simulink model "modelsim"  (R2025a)
settings: Solver=ode23t  StartTime=0.0  StopTime=10.0  MaxStep=0.01  RelTol=1e-3
undefined symbols (not defined in the file or in its folder): X, Y, Z
libraries: sm_lib x91, nesl_utility x20, slpidlib x1
(part 3 of 3)

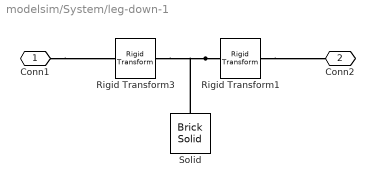
== system modelsim/System/leg-down-1 ==
  Rigid Transform1 : sm_lib/Frames and Transforms/Rigid Transform  RotationMethod=None  FollAlignAxisA=+X  BaseAlignAxisA=+Y  FollAlignAxisB=+Y  BaseAlignAxisB=+Z  RotationStandardAxis=+Z  RotationAngle=0.0  RotationAngleUnits=deg  RotationArbitraryAxis=[0 0 1]  RotationSequenceAxes=FollowerAxes  RotationSequence=XYX  RotationSequenceAngles=[0 0 0]  RotationSequenceAnglesUnits=deg  RotationMatrix=[1 0 0; 0 1 0; 0 0 1]  Quaternion=[1 0 0 0]  TranslationMethod=StandardAxis  TranslationCartesianOffset=[0 0 0]  TranslationCartesianOffsetUnits=m  TranslationStandardAxis=+X  TranslationStandardOffset=L/2  TranslationStandardOffsetUnits=m  TranslationROffset=0  TranslationROffsetUnits=m  TranslationThetaOffset=0  TranslationThetaOffsetUnits=deg  TranslationZOffset=0  TranslationZOffsetUnits=m
  Rigid Transform3 : sm_lib/Frames and Transforms/Rigid Transform  RotationMethod=None  FollAlignAxisA=+X  BaseAlignAxisA=+Y  FollAlignAxisB=+Y  BaseAlignAxisB=+Z  RotationStandardAxis=+Z  RotationAngle=0.0  RotationAngleUnits=deg  RotationArbitraryAxis=[0 0 1]  RotationSequenceAxes=FollowerAxes  RotationSequence=XYX  RotationSequenceAngles=[0 0 0]  RotationSequenceAnglesUnits=deg  RotationMatrix=[1 0 0; 0 1 0; 0 0 1]  Quaternion=[1 0 0 0]  TranslationMethod=StandardAxis  TranslationCartesianOffset=[0 0 0]  TranslationCartesianOffsetUnits=m  TranslationStandardAxis=+X  TranslationStandardOffset=L/2  TranslationStandardOffsetUnits=m  TranslationROffset=0  TranslationROffsetUnits=m  TranslationThetaOffset=0  TranslationThetaOffsetUnits=deg  TranslationZOffset=0  TranslationZOffsetUnits=m
  Solid : sm_lib/Body Elements/Brick Solid  BrickDimensions=[L H W]  BrickDimensionsUnits=m  ExportEntireGeometry=off  InertiaType=CalculateFromGeometry  BasedOnType=Density  Density=rho  DensityUnits=kg/m^3  Mass=1  MassUnits=kg  CenterOfMass=[0 0 0]  CenterOfMassUnits=m  MomentsOfInertia=[1 1 1]  MomentsOfInertiaUnits=kg*m^2  ProductsOfInertia=[0 0 0]  ProductsOfInertiaUnits=kg*m^2  GraphicType=FromGeometry  MarkerShape=Sphere  MarkerSize=10  GraphicVisPropType=SimpleVisualProperties  GraphicDiffuseColor=[0.5 0.5 0.5]  GraphicOpacity=1.0  GraphicSpecularColor=[0.5 0.5 0.5 1.0]  GraphicAmbientColor=[0.15 0.15 0.15 1.0]  GraphicEmissiveColor=[0.0 0.0 0.0 1.0]  GraphicShininess=75  DoExposeReferenceFrame=on  SerializedFrames=<Frames/>
  Conn1 : PMIOPort  Side=Left
  Conn2 : PMIOPort  Port=2  Side=Right
  connections:
  Rigid Transform1/RConn1 -- Conn2/RConn1
  Conn1/RConn1 -- Rigid Transform3/LConn1
  Rigid Transform1/LConn1 -- Solid/RConn1 -- Rigid Transform3/RConn1

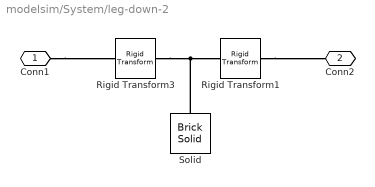
== system modelsim/System/leg-down-2 ==
  Rigid Transform1 : sm_lib/Frames and Transforms/Rigid Transform  RotationMethod=None  FollAlignAxisA=+X  BaseAlignAxisA=+Y  FollAlignAxisB=+Y  BaseAlignAxisB=+Z  RotationStandardAxis=+Z  RotationAngle=0.0  RotationAngleUnits=deg  RotationArbitraryAxis=[0 0 1]  RotationSequenceAxes=FollowerAxes  RotationSequence=XYX  RotationSequenceAngles=[0 0 0]  RotationSequenceAnglesUnits=deg  RotationMatrix=[1 0 0; 0 1 0; 0 0 1]  Quaternion=[1 0 0 0]  TranslationMethod=StandardAxis  TranslationCartesianOffset=[0 0 0]  TranslationCartesianOffsetUnits=m  TranslationStandardAxis=+X  TranslationStandardOffset=L/2  TranslationStandardOffsetUnits=m  TranslationROffset=0  TranslationROffsetUnits=m  TranslationThetaOffset=0  TranslationThetaOffsetUnits=deg  TranslationZOffset=0  TranslationZOffsetUnits=m
  Rigid Transform3 : sm_lib/Frames and Transforms/Rigid Transform  RotationMethod=None  FollAlignAxisA=+X  BaseAlignAxisA=+Y  FollAlignAxisB=+Y  BaseAlignAxisB=+Z  RotationStandardAxis=+Z  RotationAngle=0.0  RotationAngleUnits=deg  RotationArbitraryAxis=[0 0 1]  RotationSequenceAxes=FollowerAxes  RotationSequence=XYX  RotationSequenceAngles=[0 0 0]  RotationSequenceAnglesUnits=deg  RotationMatrix=[1 0 0; 0 1 0; 0 0 1]  Quaternion=[1 0 0 0]  TranslationMethod=StandardAxis  TranslationCartesianOffset=[0 0 0]  TranslationCartesianOffsetUnits=m  TranslationStandardAxis=+X  TranslationStandardOffset=L/2  TranslationStandardOffsetUnits=m  TranslationROffset=0  TranslationROffsetUnits=m  TranslationThetaOffset=0  TranslationThetaOffsetUnits=deg  TranslationZOffset=0  TranslationZOffsetUnits=m
  Solid : sm_lib/Body Elements/Brick Solid  BrickDimensions=[L H W]  BrickDimensionsUnits=m  ExportEntireGeometry=off  InertiaType=CalculateFromGeometry  BasedOnType=Density  Density=rho  DensityUnits=kg/m^3  Mass=1  MassUnits=kg  CenterOfMass=[0 0 0]  CenterOfMassUnits=m  MomentsOfInertia=[1 1 1]  MomentsOfInertiaUnits=kg*m^2  ProductsOfInertia=[0 0 0]  ProductsOfInertiaUnits=kg*m^2  GraphicType=FromGeometry  MarkerShape=Sphere  MarkerSize=10  GraphicVisPropType=SimpleVisualProperties  GraphicDiffuseColor=[0.5 0.5 0.5]  GraphicOpacity=1.0  GraphicSpecularColor=[0.5 0.5 0.5 1.0]  GraphicAmbientColor=[0.15 0.15 0.15 1.0]  GraphicEmissiveColor=[0.0 0.0 0.0 1.0]  GraphicShininess=75  DoExposeReferenceFrame=on  SerializedFrames=<Frames/>
  Conn1 : PMIOPort  Side=Left
  Conn2 : PMIOPort  Port=2  Side=Right
  connections:
  Rigid Transform3/RConn1 -- Solid/RConn1 -- Rigid Transform1/LConn1
  Conn1/RConn1 -- Rigid Transform3/LConn1
  Rigid Transform1/RConn1 -- Conn2/RConn1

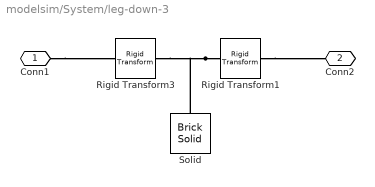
== system modelsim/System/leg-down-3 ==
  Rigid Transform1 : sm_lib/Frames and Transforms/Rigid Transform  RotationMethod=None  FollAlignAxisA=+X  BaseAlignAxisA=+Y  FollAlignAxisB=+Y  BaseAlignAxisB=+Z  RotationStandardAxis=+Z  RotationAngle=0.0  RotationAngleUnits=deg  RotationArbitraryAxis=[0 0 1]  RotationSequenceAxes=FollowerAxes  RotationSequence=XYX  RotationSequenceAngles=[0 0 0]  RotationSequenceAnglesUnits=deg  RotationMatrix=[1 0 0; 0 1 0; 0 0 1]  Quaternion=[1 0 0 0]  TranslationMethod=StandardAxis  TranslationCartesianOffset=[0 0 0]  TranslationCartesianOffsetUnits=m  TranslationStandardAxis=+X  TranslationStandardOffset=L/2  TranslationStandardOffsetUnits=m  TranslationROffset=0  TranslationROffsetUnits=m  TranslationThetaOffset=0  TranslationThetaOffsetUnits=deg  TranslationZOffset=0  TranslationZOffsetUnits=m
  Rigid Transform3 : sm_lib/Frames and Transforms/Rigid Transform  RotationMethod=None  FollAlignAxisA=+X  BaseAlignAxisA=+Y  FollAlignAxisB=+Y  BaseAlignAxisB=+Z  RotationStandardAxis=+Z  RotationAngle=0.0  RotationAngleUnits=deg  RotationArbitraryAxis=[0 0 1]  RotationSequenceAxes=FollowerAxes  RotationSequence=XYX  RotationSequenceAngles=[0 0 0]  RotationSequenceAnglesUnits=deg  RotationMatrix=[1 0 0; 0 1 0; 0 0 1]  Quaternion=[1 0 0 0]  TranslationMethod=StandardAxis  TranslationCartesianOffset=[0 0 0]  TranslationCartesianOffsetUnits=m  TranslationStandardAxis=+X  TranslationStandardOffset=L/2  TranslationStandardOffsetUnits=m  TranslationROffset=0  TranslationROffsetUnits=m  TranslationThetaOffset=0  TranslationThetaOffsetUnits=deg  TranslationZOffset=0  TranslationZOffsetUnits=m
  Solid : sm_lib/Body Elements/Brick Solid  BrickDimensions=[L H W]  BrickDimensionsUnits=m  ExportEntireGeometry=off  InertiaType=CalculateFromGeometry  BasedOnType=Density  Density=rho  DensityUnits=kg/m^3  Mass=1  MassUnits=kg  CenterOfMass=[0 0 0]  CenterOfMassUnits=m  MomentsOfInertia=[1 1 1]  MomentsOfInertiaUnits=kg*m^2  ProductsOfInertia=[0 0 0]  ProductsOfInertiaUnits=kg*m^2  GraphicType=FromGeometry  MarkerShape=Sphere  MarkerSize=10  GraphicVisPropType=SimpleVisualProperties  GraphicDiffuseColor=[0.5 0.5 0.5]  GraphicOpacity=1.0  GraphicSpecularColor=[0.5 0.5 0.5 1.0]  GraphicAmbientColor=[0.15 0.15 0.15 1.0]  GraphicEmissiveColor=[0.0 0.0 0.0 1.0]  GraphicShininess=75  DoExposeReferenceFrame=on  SerializedFrames=<Frames/>
  Conn1 : PMIOPort  Side=Left
  Conn2 : PMIOPort  Port=2  Side=Right
  connections:
  Rigid Transform1/RConn1 -- Conn2/RConn1
  Conn1/RConn1 -- Rigid Transform3/LConn1
  Rigid Transform1/LConn1 -- Solid/RConn1 -- Rigid Transform3/RConn1

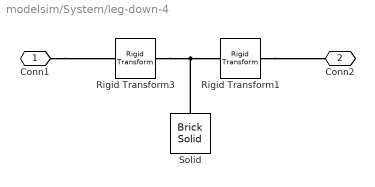
== system modelsim/System/leg-down-4 ==
  Rigid Transform1 : sm_lib/Frames and Transforms/Rigid Transform  RotationMethod=None  FollAlignAxisA=+X  BaseAlignAxisA=+Y  FollAlignAxisB=+Y  BaseAlignAxisB=+Z  RotationStandardAxis=+Z  RotationAngle=0.0  RotationAngleUnits=deg  RotationArbitraryAxis=[0 0 1]  RotationSequenceAxes=FollowerAxes  RotationSequence=XYX  RotationSequenceAngles=[0 0 0]  RotationSequenceAnglesUnits=deg  RotationMatrix=[1 0 0; 0 1 0; 0 0 1]  Quaternion=[1 0 0 0]  TranslationMethod=StandardAxis  TranslationCartesianOffset=[0 0 0]  TranslationCartesianOffsetUnits=m  TranslationStandardAxis=+X  TranslationStandardOffset=L/2  TranslationStandardOffsetUnits=m  TranslationROffset=0  TranslationROffsetUnits=m  TranslationThetaOffset=0  TranslationThetaOffsetUnits=deg  TranslationZOffset=0  TranslationZOffsetUnits=m
  Rigid Transform3 : sm_lib/Frames and Transforms/Rigid Transform  RotationMethod=None  FollAlignAxisA=+X  BaseAlignAxisA=+Y  FollAlignAxisB=+Y  BaseAlignAxisB=+Z  RotationStandardAxis=+Z  RotationAngle=0.0  RotationAngleUnits=deg  RotationArbitraryAxis=[0 0 1]  RotationSequenceAxes=FollowerAxes  RotationSequence=XYX  RotationSequenceAngles=[0 0 0]  RotationSequenceAnglesUnits=deg  RotationMatrix=[1 0 0; 0 1 0; 0 0 1]  Quaternion=[1 0 0 0]  TranslationMethod=StandardAxis  TranslationCartesianOffset=[0 0 0]  TranslationCartesianOffsetUnits=m  TranslationStandardAxis=+X  TranslationStandardOffset=L/2  TranslationStandardOffsetUnits=m  TranslationROffset=0  TranslationROffsetUnits=m  TranslationThetaOffset=0  TranslationThetaOffsetUnits=deg  TranslationZOffset=0  TranslationZOffsetUnits=m
  Solid : sm_lib/Body Elements/Brick Solid  BrickDimensions=[L H W]  BrickDimensionsUnits=m  ExportEntireGeometry=off  InertiaType=CalculateFromGeometry  BasedOnType=Density  Density=rho  DensityUnits=kg/m^3  Mass=1  MassUnits=kg  CenterOfMass=[0 0 0]  CenterOfMassUnits=m  MomentsOfInertia=[1 1 1]  MomentsOfInertiaUnits=kg*m^2  ProductsOfInertia=[0 0 0]  ProductsOfInertiaUnits=kg*m^2  GraphicType=FromGeometry  MarkerShape=Sphere  MarkerSize=10  GraphicVisPropType=SimpleVisualProperties  GraphicDiffuseColor=[0.5 0.5 0.5]  GraphicOpacity=1.0  GraphicSpecularColor=[0.5 0.5 0.5 1.0]  GraphicAmbientColor=[0.15 0.15 0.15 1.0]  GraphicEmissiveColor=[0.0 0.0 0.0 1.0]  GraphicShininess=75  DoExposeReferenceFrame=on  SerializedFrames=<Frames/>
  Conn1 : PMIOPort  Side=Left
  Conn2 : PMIOPort  Port=2  Side=Right
  connections:
  Rigid Transform3/RConn1 -- Solid/RConn1 -- Rigid Transform1/LConn1
  Conn1/RConn1 -- Rigid Transform3/LConn1
  Rigid Transform1/RConn1 -- Conn2/RConn1

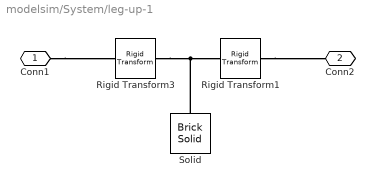
== system modelsim/System/leg-up-1 ==
  Rigid Transform1 : sm_lib/Frames and Transforms/Rigid Transform  RotationMethod=None  FollAlignAxisA=+X  BaseAlignAxisA=+Y  FollAlignAxisB=+Y  BaseAlignAxisB=+Z  RotationStandardAxis=+Z  RotationAngle=0.0  RotationAngleUnits=deg  RotationArbitraryAxis=[0 0 1]  RotationSequenceAxes=FollowerAxes  RotationSequence=XYX  RotationSequenceAngles=[0 0 0]  RotationSequenceAnglesUnits=deg  RotationMatrix=[1 0 0; 0 1 0; 0 0 1]  Quaternion=[1 0 0 0]  TranslationMethod=StandardAxis  TranslationCartesianOffset=[0 0 0]  TranslationCartesianOffsetUnits=m  TranslationStandardAxis=+X  TranslationStandardOffset=L/2  TranslationStandardOffsetUnits=m  TranslationROffset=0  TranslationROffsetUnits=m  TranslationThetaOffset=0  TranslationThetaOffsetUnits=deg  TranslationZOffset=0  TranslationZOffsetUnits=m
  Rigid Transform3 : sm_lib/Frames and Transforms/Rigid Transform  RotationMethod=None  FollAlignAxisA=+X  BaseAlignAxisA=+Y  FollAlignAxisB=+Y  BaseAlignAxisB=+Z  RotationStandardAxis=+Z  RotationAngle=0.0  RotationAngleUnits=deg  RotationArbitraryAxis=[0 0 1]  RotationSequenceAxes=FollowerAxes  RotationSequence=XYX  RotationSequenceAngles=[0 0 0]  RotationSequenceAnglesUnits=deg  RotationMatrix=[1 0 0; 0 1 0; 0 0 1]  Quaternion=[1 0 0 0]  TranslationMethod=StandardAxis  TranslationCartesianOffset=[0 0 0]  TranslationCartesianOffsetUnits=m  TranslationStandardAxis=+X  TranslationStandardOffset=L/2  TranslationStandardOffsetUnits=m  TranslationROffset=0  TranslationROffsetUnits=m  TranslationThetaOffset=0  TranslationThetaOffsetUnits=deg  TranslationZOffset=0  TranslationZOffsetUnits=m
  Solid : sm_lib/Body Elements/Brick Solid  BrickDimensions=[L H W]  BrickDimensionsUnits=m  ExportEntireGeometry=off  InertiaType=CalculateFromGeometry  BasedOnType=Density  Density=rho  DensityUnits=kg/m^3  Mass=1  MassUnits=kg  CenterOfMass=[0 0 0]  CenterOfMassUnits=m  MomentsOfInertia=[1 1 1]  MomentsOfInertiaUnits=kg*m^2  ProductsOfInertia=[0 0 0]  ProductsOfInertiaUnits=kg*m^2  GraphicType=FromGeometry  MarkerShape=Sphere  MarkerSize=10  GraphicVisPropType=SimpleVisualProperties  GraphicDiffuseColor=[0.5 0.5 0.5]  GraphicOpacity=1.0  GraphicSpecularColor=[0.5 0.5 0.5 1.0]  GraphicAmbientColor=[0.15 0.15 0.15 1.0]  GraphicEmissiveColor=[0.0 0.0 0.0 1.0]  GraphicShininess=75  DoExposeReferenceFrame=on  SerializedFrames=<Frames/>
  Conn1 : PMIOPort  Side=Left
  Conn2 : PMIOPort  Port=2  Side=Right
  connections:
  Solid/RConn1 -- Rigid Transform3/RConn1 -- Rigid Transform1/LConn1
  Conn1/RConn1 -- Rigid Transform3/LConn1
  Rigid Transform1/RConn1 -- Conn2/RConn1

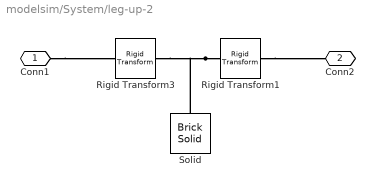
== system modelsim/System/leg-up-2 ==
  Rigid Transform1 : sm_lib/Frames and Transforms/Rigid Transform  RotationMethod=None  FollAlignAxisA=+X  BaseAlignAxisA=+Y  FollAlignAxisB=+Y  BaseAlignAxisB=+Z  RotationStandardAxis=+Z  RotationAngle=0.0  RotationAngleUnits=deg  RotationArbitraryAxis=[0 0 1]  RotationSequenceAxes=FollowerAxes  RotationSequence=XYX  RotationSequenceAngles=[0 0 0]  RotationSequenceAnglesUnits=deg  RotationMatrix=[1 0 0; 0 1 0; 0 0 1]  Quaternion=[1 0 0 0]  TranslationMethod=StandardAxis  TranslationCartesianOffset=[0 0 0]  TranslationCartesianOffsetUnits=m  TranslationStandardAxis=+X  TranslationStandardOffset=L/2  TranslationStandardOffsetUnits=m  TranslationROffset=0  TranslationROffsetUnits=m  TranslationThetaOffset=0  TranslationThetaOffsetUnits=deg  TranslationZOffset=0  TranslationZOffsetUnits=m
  Rigid Transform3 : sm_lib/Frames and Transforms/Rigid Transform  RotationMethod=None  FollAlignAxisA=+X  BaseAlignAxisA=+Y  FollAlignAxisB=+Y  BaseAlignAxisB=+Z  RotationStandardAxis=+Z  RotationAngle=0.0  RotationAngleUnits=deg  RotationArbitraryAxis=[0 0 1]  RotationSequenceAxes=FollowerAxes  RotationSequence=XYX  RotationSequenceAngles=[0 0 0]  RotationSequenceAnglesUnits=deg  RotationMatrix=[1 0 0; 0 1 0; 0 0 1]  Quaternion=[1 0 0 0]  TranslationMethod=StandardAxis  TranslationCartesianOffset=[0 0 0]  TranslationCartesianOffsetUnits=m  TranslationStandardAxis=+X  TranslationStandardOffset=L/2  TranslationStandardOffsetUnits=m  TranslationROffset=0  TranslationROffsetUnits=m  TranslationThetaOffset=0  TranslationThetaOffsetUnits=deg  TranslationZOffset=0  TranslationZOffsetUnits=m
  Solid : sm_lib/Body Elements/Brick Solid  BrickDimensions=[L H W]  BrickDimensionsUnits=m  ExportEntireGeometry=off  InertiaType=CalculateFromGeometry  BasedOnType=Density  Density=rho  DensityUnits=kg/m^3  Mass=1  MassUnits=kg  CenterOfMass=[0 0 0]  CenterOfMassUnits=m  MomentsOfInertia=[1 1 1]  MomentsOfInertiaUnits=kg*m^2  ProductsOfInertia=[0 0 0]  ProductsOfInertiaUnits=kg*m^2  GraphicType=FromGeometry  MarkerShape=Sphere  MarkerSize=10  GraphicVisPropType=SimpleVisualProperties  GraphicDiffuseColor=[0.5 0.5 0.5]  GraphicOpacity=1.0  GraphicSpecularColor=[0.5 0.5 0.5 1.0]  GraphicAmbientColor=[0.15 0.15 0.15 1.0]  GraphicEmissiveColor=[0.0 0.0 0.0 1.0]  GraphicShininess=75  DoExposeReferenceFrame=on  SerializedFrames=<Frames/>
  Conn1 : PMIOPort  Side=Left
  Conn2 : PMIOPort  Port=2  Side=Right
  connections:
  Rigid Transform1/RConn1 -- Conn2/RConn1
  Conn1/RConn1 -- Rigid Transform3/LConn1
  Rigid Transform1/LConn1 -- Solid/RConn1 -- Rigid Transform3/RConn1

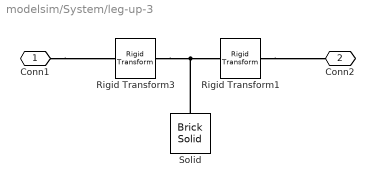
== system modelsim/System/leg-up-3 ==
  Rigid Transform1 : sm_lib/Frames and Transforms/Rigid Transform  RotationMethod=None  FollAlignAxisA=+X  BaseAlignAxisA=+Y  FollAlignAxisB=+Y  BaseAlignAxisB=+Z  RotationStandardAxis=+Z  RotationAngle=0.0  RotationAngleUnits=deg  RotationArbitraryAxis=[0 0 1]  RotationSequenceAxes=FollowerAxes  RotationSequence=XYX  RotationSequenceAngles=[0 0 0]  RotationSequenceAnglesUnits=deg  RotationMatrix=[1 0 0; 0 1 0; 0 0 1]  Quaternion=[1 0 0 0]  TranslationMethod=StandardAxis  TranslationCartesianOffset=[0 0 0]  TranslationCartesianOffsetUnits=m  TranslationStandardAxis=+X  TranslationStandardOffset=L/2  TranslationStandardOffsetUnits=m  TranslationROffset=0  TranslationROffsetUnits=m  TranslationThetaOffset=0  TranslationThetaOffsetUnits=deg  TranslationZOffset=0  TranslationZOffsetUnits=m
  Rigid Transform3 : sm_lib/Frames and Transforms/Rigid Transform  RotationMethod=None  FollAlignAxisA=+X  BaseAlignAxisA=+Y  FollAlignAxisB=+Y  BaseAlignAxisB=+Z  RotationStandardAxis=+Z  RotationAngle=0.0  RotationAngleUnits=deg  RotationArbitraryAxis=[0 0 1]  RotationSequenceAxes=FollowerAxes  RotationSequence=XYX  RotationSequenceAngles=[0 0 0]  RotationSequenceAnglesUnits=deg  RotationMatrix=[1 0 0; 0 1 0; 0 0 1]  Quaternion=[1 0 0 0]  TranslationMethod=StandardAxis  TranslationCartesianOffset=[0 0 0]  TranslationCartesianOffsetUnits=m  TranslationStandardAxis=+X  TranslationStandardOffset=L/2  TranslationStandardOffsetUnits=m  TranslationROffset=0  TranslationROffsetUnits=m  TranslationThetaOffset=0  TranslationThetaOffsetUnits=deg  TranslationZOffset=0  TranslationZOffsetUnits=m
  Solid : sm_lib/Body Elements/Brick Solid  BrickDimensions=[L H W]  BrickDimensionsUnits=m  ExportEntireGeometry=off  InertiaType=CalculateFromGeometry  BasedOnType=Density  Density=rho  DensityUnits=kg/m^3  Mass=1  MassUnits=kg  CenterOfMass=[0 0 0]  CenterOfMassUnits=m  MomentsOfInertia=[1 1 1]  MomentsOfInertiaUnits=kg*m^2  ProductsOfInertia=[0 0 0]  ProductsOfInertiaUnits=kg*m^2  GraphicType=FromGeometry  MarkerShape=Sphere  MarkerSize=10  GraphicVisPropType=SimpleVisualProperties  GraphicDiffuseColor=[0.5 0.5 0.5]  GraphicOpacity=1.0  GraphicSpecularColor=[0.5 0.5 0.5 1.0]  GraphicAmbientColor=[0.15 0.15 0.15 1.0]  GraphicEmissiveColor=[0.0 0.0 0.0 1.0]  GraphicShininess=75  DoExposeReferenceFrame=on  SerializedFrames=<Frames/>
  Conn1 : PMIOPort  Side=Left
  Conn2 : PMIOPort  Port=2  Side=Right
  connections:
  Solid/RConn1 -- Rigid Transform3/RConn1 -- Rigid Transform1/LConn1
  Conn1/RConn1 -- Rigid Transform3/LConn1
  Rigid Transform1/RConn1 -- Conn2/RConn1

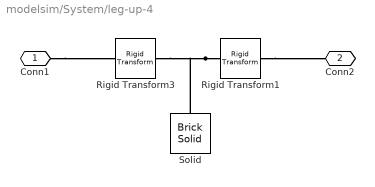
== system modelsim/System/leg-up-4 ==
  Rigid Transform1 : sm_lib/Frames and Transforms/Rigid Transform  RotationMethod=None  FollAlignAxisA=+X  BaseAlignAxisA=+Y  FollAlignAxisB=+Y  BaseAlignAxisB=+Z  RotationStandardAxis=+Z  RotationAngle=0.0  RotationAngleUnits=deg  RotationArbitraryAxis=[0 0 1]  RotationSequenceAxes=FollowerAxes  RotationSequence=XYX  RotationSequenceAngles=[0 0 0]  RotationSequenceAnglesUnits=deg  RotationMatrix=[1 0 0; 0 1 0; 0 0 1]  Quaternion=[1 0 0 0]  TranslationMethod=StandardAxis  TranslationCartesianOffset=[0 0 0]  TranslationCartesianOffsetUnits=m  TranslationStandardAxis=+X  TranslationStandardOffset=L/2  TranslationStandardOffsetUnits=m  TranslationROffset=0  TranslationROffsetUnits=m  TranslationThetaOffset=0  TranslationThetaOffsetUnits=deg  TranslationZOffset=0  TranslationZOffsetUnits=m
  Rigid Transform3 : sm_lib/Frames and Transforms/Rigid Transform  RotationMethod=None  FollAlignAxisA=+X  BaseAlignAxisA=+Y  FollAlignAxisB=+Y  BaseAlignAxisB=+Z  RotationStandardAxis=+Z  RotationAngle=0.0  RotationAngleUnits=deg  RotationArbitraryAxis=[0 0 1]  RotationSequenceAxes=FollowerAxes  RotationSequence=XYX  RotationSequenceAngles=[0 0 0]  RotationSequenceAnglesUnits=deg  RotationMatrix=[1 0 0; 0 1 0; 0 0 1]  Quaternion=[1 0 0 0]  TranslationMethod=StandardAxis  TranslationCartesianOffset=[0 0 0]  TranslationCartesianOffsetUnits=m  TranslationStandardAxis=+X  TranslationStandardOffset=L/2  TranslationStandardOffsetUnits=m  TranslationROffset=0  TranslationROffsetUnits=m  TranslationThetaOffset=0  TranslationThetaOffsetUnits=deg  TranslationZOffset=0  TranslationZOffsetUnits=m
  Solid : sm_lib/Body Elements/Brick Solid  BrickDimensions=[L H W]  BrickDimensionsUnits=m  ExportEntireGeometry=off  InertiaType=CalculateFromGeometry  BasedOnType=Density  Density=rho  DensityUnits=kg/m^3  Mass=1  MassUnits=kg  CenterOfMass=[0 0 0]  CenterOfMassUnits=m  MomentsOfInertia=[1 1 1]  MomentsOfInertiaUnits=kg*m^2  ProductsOfInertia=[0 0 0]  ProductsOfInertiaUnits=kg*m^2  GraphicType=FromGeometry  MarkerShape=Sphere  MarkerSize=10  GraphicVisPropType=SimpleVisualProperties  GraphicDiffuseColor=[0.5 0.5 0.5]  GraphicOpacity=1.0  GraphicSpecularColor=[0.5 0.5 0.5 1.0]  GraphicAmbientColor=[0.15 0.15 0.15 1.0]  GraphicEmissiveColor=[0.0 0.0 0.0 1.0]  GraphicShininess=75  DoExposeReferenceFrame=on  SerializedFrames=<Frames/>
  Conn1 : PMIOPort  Side=Left
  Conn2 : PMIOPort  Port=2  Side=Right
  connections:
  Rigid Transform1/RConn1 -- Conn2/RConn1
  Conn1/RConn1 -- Rigid Transform3/LConn1
  Rigid Transform1/LConn1 -- Solid/RConn1 -- Rigid Transform3/RConn1

== matlab function modelsim/MATLAB Function1 ==
  data: L output; phi0 output; phi1 input; xdot output; phi4 input; phi1dot input; phi4dot input
function [L,phi0,xdot] = vmcX(phi1,phi4,phi1dot,phi4dot)
%vmcX
%    [L,PHI0,XDOT] = vmcX(PHI1,PHI4,PHI1DOT,PHI4DOT)

%    This function was generated by the Symbolic Math Toolbox version 25.1.
%    2025-12-08 16:42:02

t2 = cos(phi1);
t3 = cos(phi4);
t4 = sin(phi1);
t5 = sin(phi4);
t6 = t2.*(3.0./2.0e+1);
t7 = t3.*(3.0./2.0e+1);
t8 = t4.*(3.0./2.0e+1);
t9 = t5.*(3.0./2.0e+1);
t12 = t4.*1.5e-1i;
t13 = t5.*1.5e-1i;
t15 = t2.*(8.1e+1./1.0e+3);
t16 = t3.*(8.1e+1./1.0e+3);
t17 = t4.*(8.1e+1./1.0e+3);
t18 = t5.*(8.1e+1./1.0e+3);
t21 = t4.*8.1e-2i;
t22 = t5.*8.1e-2i;
t10 = -t6;
t11 = -t9;
t14 = -t12;
t19 = -t15;
t20 = -t18;
t23 = -t21;
t24 = t8+t11;
t26 = t7+t10+3.0./2.0e+1;
t28 = t17+t20;
t30 = t16+t19+8.1e+1./1.0e+3;
t25 = t24.^2;
t27 = t26.^2;
t29 = t28.^2;
t31 = t30.^2;
t32 = t25+t27;
t33 = t32.^2;
t34 = -t33;
t35 = t29+t31+t34;
t36 = sqrt(t35);
t37 = t36.*1i;
t38 = t22+t23+t30+t32+t37;
t39 = angle(t38);
t40 = t39.*2.0;
t41 = -t40;
t42 = cos(t40);
t43 = sin(t40);
t44 = phi1+t41;
t45 = phi4+t41;
t48 = t42.*(2.7e+1./1.0e+2);
t49 = t43.*(2.7e+1./1.0e+2);
t51 = t43.*2.7e-1i;
t46 = sin(t44);
t47 = sin(t45);
t50 = -t48;
t52 = -t51;
t53 = t8+t49;
t55 = t6+t48-3.0./4.0e+1;
t54 = t53.^2;
t56 = t55.^2;
t57 = t12+t51+t55;
t64 = t13+t14+t26+t50+t52;
t58 = angle(t57);
t59 = t54+t56;
t65 = angle(t64);
t60 = -t58;
t63 = 1.0./sqrt(t59);
L = 1.0./t63;
if nargout > 1
    phi0 = t58;
end
if nargout > 2
    t66 = -t65;
    t61 = phi1+t60;
    t62 = phi4+t60;
    t67 = phi1+t66;
    t68 = phi4+t66;
    t71 = t40+t60;
    t74 = t40+t66;
    t77 = t60+t65;
    t69 = sin(t67);
    t70 = sin(t68);
    t72 = cos(t71);
    t73 = sin(t71);
    t75 = sin(t74);
    t78 = cos(t77);
    t79 = sin(t77);
    t76 = 1.0./t75;
    xdot = [phi1dot.*(sin(t61).*(-3.0./2.0e+1)+t46.*t76.*t79.*(3.0./2.0e+1)+t69.*t73.*t76.*(3.0./2.0e+1))-phi4dot.*(sin(t62).*(3.0./2.0e+1)+t47.*t76.*t79.*(3.0./2.0e+1)+t70.*t73.*t76.*(3.0./2.0e+1));-phi1dot.*t63.*(cos(t61).*(-3.0./2.0e+1)+t46.*t76.*t78.*(3.0./2.0e+1)+t69.*t72.*t76.*(3.0./2.0e+1))+phi4dot.*t63.*(cos(t62).*(3.0./2.0e+1)+t47.*t76.*t78.*(3.0./2.0e+1)+t70.*t72.*t76.*(3.0./2.0e+1))];
end
end

== matlab function modelsim/MATLAB Function ==
  data: F input; T output; Tp input; phi1 input; phi4 input
function T = vmcT(F,Tp,phi1,phi4)
%vmcT
%    T = vmcT(F,Tp,PHI1,PHI4)

%    This function was generated by the Symbolic Math Toolbox version 25.1.
%    2025-12-08 15:34:32

t2 = cos(phi1);
t3 = cos(phi4);
t4 = sin(phi1);
t5 = sin(phi4);
t6 = t2.*(3.0./2.0e+1);
t7 = t3.*(3.0./2.0e+1);
t8 = t4.*(3.0./2.0e+1);
t9 = t5.*(3.0./2.0e+1);
t12 = t4.*1.5e-1i;
t13 = t5.*1.5e-1i;
t15 = t2.*(8.1e+1./1.0e+3);
t16 = t3.*(8.1e+1./1.0e+3);
t17 = t4.*(8.1e+1./1.0e+3);
t18 = t5.*(8.1e+1./1.0e+3);
t21 = t4.*8.1e-2i;
t22 = t5.*8.1e-2i;
t10 = -t6;
t11 = -t9;
t14 = -t12;
t19 = -t15;
t20 = -t18;
t23 = -t21;
t24 = t8+t11;
t26 = t7+t10+3.0./2.0e+1;
t28 = t17+t20;
t30 = t16+t19+8.1e+1./1.0e+3;
t25 = t24.^2;
t27 = t26.^2;
t29 = t28.^2;
t31 = t30.^2;
t32 = t25+t27;
t33 = t32.^2;
t34 = -t33;
t35 = t29+t31+t34;
t36 = sqrt(t35);
t37 = t36.*1i;
t38 = t22+t23+t30+t32+t37;
t39 = angle(t38);
t40 = t39.*2.0;
t41 = -t40;
t42 = cos(t40);
t43 = sin(t40);
t44 = phi1+t41;
t45 = phi4+t41;
t48 = t42.*(2.7e+1./1.0e+2);
t49 = t43.*(2.7e+1./1.0e+2);
t51 = t43.*2.7e-1i;
t46 = sin(t44);
t47 = sin(t45);
t50 = -t48;
t52 = -t51;
t53 = t8+t49;
t55 = t6+t48-3.0./4.0e+1;
t54 = t53.^2;
t56 = t55.^2;
t57 = t12+t51+t55;
t64 = t13+t14+t26+t50+t52;
t58 = angle(t57);
t59 = t54+t56;
t65 = angle(t64);
t60 = -t58;
t63 = 1.0./sqrt(t59);
t66 = -t65;
t61 = phi1+t60;
t62 = phi4+t60;
t67 = phi1+t66;
t68 = phi4+t66;
t71 = t40+t60;
t74 = t40+t66;
t77 = t60+t65;
t69 = sin(t67);
t70 = sin(t68);
t72 = cos(t71);
t73 = sin(t71);
t75 = sin(t74);
t78 = cos(t77);
t79 = sin(t77);
t76 = 1.0./t75;
T = [F.*(sin(t61).*(-3.0./2.0e+1)+t46.*t76.*t79.*(3.0./2.0e+1)+t69.*t73.*t76.*(3.0./2.0e+1))-Tp.*t63.*(cos(t61).*(-3.0./2.0e+1)+t46.*t76.*t78.*(3.0./2.0e+1)+t69.*t72.*t76.*(3.0./2.0e+1));-F.*(sin(t62).*(3.0./2.0e+1)+t47.*t76.*t79.*(3.0./2.0e+1)+t70.*t73.*t76.*(3.0./2.0e+1))+Tp.*t63.*(cos(t62).*(3.0./2.0e+1)+t47.*t76.*t78.*(3.0./2.0e+1)+t70.*t72.*t76.*(3.0./2.0e+1))];
end

== matlab function modelsim/MATLAB Function2 ==
  data: Lval input; Kfit output
function Kfit = kfun(Lval)
%KFUN
%    Kfit = KFUN(Lval)

%    This function was generated by the Symbolic Math Toolbox version 25.1.
%    2025-12-08 12:10:09

t2 = Lval.^2;
t3 = Lval.^3;
mt1 = [Lval.*(-2.358484958447678e+2)+t2.*4.883859267029833e+2-t3.*4.197090716510888e+2-6.581551887761631];
mt2 = [Lval.*2.209681597124775e+1-t2.*9.994239621274812e+1+t3.*1.140978245006587e+2+5.168827761637286];
mt3 = [Lval.*(-1.055401859922007e+1)-t2.*7.215491684985574+t3.*1.159102876879173e+1-1.836023120103903];
mt4 = [Lval.*(-6.731520694019014e-1)+t2.*1.650634272126259-t3.*1.969773866086712+8.962408876058987e-1];
mt5 = [Lval.*(-1.251824460139937)+t2.*3.213004812895351-t3.*3.062426392413356-2.42388801840402e-1];
mt6 = [Lval.*(-8.338686274219771e-1)+t2.*1.427850383599749-t3.*1.021333899788594+2.61416634958663e-1];
mt7 = [Lval.*(-5.93423557383092)+t2.*1.472636688020171e+1-t3.*1.389021063875579e+1-1.291965322245365];
mt8 = [Lval.*(-4.279957246429905)+t2.*7.518704300149749-t3.*5.532520226555231+1.322153918137459];
mt9 = [Lval.*1.206967690398176e-1-t2.*2.106359562793197e-1+t3.*1.539064048025308e-1-3.729754493023236e-2];
mt10 = [Lval.*(-7.084838245974999e-2)+t2.*1.742629615013347e-1-t3.*1.604231063278101e-1-1.960314368955645e-2];
mt11 = [Lval.*6.678869437640343-t2.*1.167254716785922e+1+t3.*8.542517461227344-2.062447068741418];
mt12 = [Lval.*(-3.918289688474408)+t2.*9.639880814665997-t3.*8.876153431568705-1.080582612172419];
Kfit = reshape([mt1,mt2,mt3,mt4,mt5,mt6,mt7,mt8,mt9,mt10,mt11,mt12],2,6);
end

== matlab function modelsim/MATLAB Function3 ==
  data: L output; phi0 output; phi1 input; xdot output; phi4 input; phi1dot input; phi4dot input
function [L,phi0,xdot] = vmcX(phi1,phi4,phi1dot,phi4dot)
%vmcX
%    [L,PHI0,XDOT] = vmcX(PHI1,PHI4,PHI1DOT,PHI4DOT)

%    This function was generated by the Symbolic Math Toolbox version 25.1.
%    2025-12-08 16:42:02

t2 = cos(phi1);
t3 = cos(phi4);
t4 = sin(phi1);
t5 = sin(phi4);
t6 = t2.*(3.0./2.0e+1);
t7 = t3.*(3.0./2.0e+1);
t8 = t4.*(3.0./2.0e+1);
t9 = t5.*(3.0./2.0e+1);
t12 = t4.*1.5e-1i;
t13 = t5.*1.5e-1i;
t15 = t2.*(8.1e+1./1.0e+3);
t16 = t3.*(8.1e+1./1.0e+3);
t17 = t4.*(8.1e+1./1.0e+3);
t18 = t5.*(8.1e+1./1.0e+3);
t21 = t4.*8.1e-2i;
t22 = t5.*8.1e-2i;
t10 = -t6;
t11 = -t9;
t14 = -t12;
t19 = -t15;
t20 = -t18;
t23 = -t21;
t24 = t8+t11;
t26 = t7+t10+3.0./2.0e+1;
t28 = t17+t20;
t30 = t16+t19+8.1e+1./1.0e+3;
t25 = t24.^2;
t27 = t26.^2;
t29 = t28.^2;
t31 = t30.^2;
t32 = t25+t27;
t33 = t32.^2;
t34 = -t33;
t35 = t29+t31+t34;
t36 = sqrt(t35);
t37 = t36.*1i;
t38 = t22+t23+t30+t32+t37;
t39 = angle(t38);
t40 = t39.*2.0;
t41 = -t40;
t42 = cos(t40);
t43 = sin(t40);
t44 = phi1+t41;
t45 = phi4+t41;
t48 = t42.*(2.7e+1./1.0e+2);
t49 = t43.*(2.7e+1./1.0e+2);
t51 = t43.*2.7e-1i;
t46 = sin(t44);
t47 = sin(t45);
t50 = -t48;
t52 = -t51;
t53 = t8+t49;
t55 = t6+t48-3.0./4.0e+1;
t54 = t53.^2;
t56 = t55.^2;
t57 = t12+t51+t55;
t64 = t13+t14+t26+t50+t52;
t58 = angle(t57);
t59 = t54+t56;
t65 = angle(t64);
t60 = -t58;
t63 = 1.0./sqrt(t59);
L = 1.0./t63;
if nargout > 1
    phi0 = t58;
end
if nargout > 2
    t66 = -t65;
    t61 = phi1+t60;
    t62 = phi4+t60;
    t67 = phi1+t66;
    t68 = phi4+t66;
    t71 = t40+t60;
    t74 = t40+t66;
    t77 = t60+t65;
    t69 = sin(t67);
    t70 = sin(t68);
    t72 = cos(t71);
    t73 = sin(t71);
    t75 = sin(t74);
    t78 = cos(t77);
    t79 = sin(t77);
    t76 = 1.0./t75;
    xdot = [phi1dot.*(sin(t61).*(-3.0./2.0e+1)+t46.*t76.*t79.*(3.0./2.0e+1)+t69.*t73.*t76.*(3.0./2.0e+1))-phi4dot.*(sin(t62).*(3.0./2.0e+1)+t47.*t76.*t79.*(3.0./2.0e+1)+t70.*t73.*t76.*(3.0./2.0e+1));-phi1dot.*t63.*(cos(t61).*(-3.0./2.0e+1)+t46.*t76.*t78.*(3.0./2.0e+1)+t69.*t72.*t76.*(3.0./2.0e+1))+phi4dot.*t63.*(cos(t62).*(3.0./2.0e+1)+t47.*t76.*t78.*(3.0./2.0e+1)+t70.*t72.*t76.*(3.0./2.0e+1))];
end
end

== matlab function modelsim/MATLAB Function4 ==
  data: F input; T output; Tp input; phi1 input; phi4 input
function T = vmcT(F,Tp,phi1,phi4)
%vmcT
%    T = vmcT(F,Tp,PHI1,PHI4)

%    This function was generated by the Symbolic Math Toolbox version 25.1.
%    2025-12-08 15:34:32

t2 = cos(phi1);
t3 = cos(phi4);
t4 = sin(phi1);
t5 = sin(phi4);
t6 = t2.*(3.0./2.0e+1);
t7 = t3.*(3.0./2.0e+1);
t8 = t4.*(3.0./2.0e+1);
t9 = t5.*(3.0./2.0e+1);
t12 = t4.*1.5e-1i;
t13 = t5.*1.5e-1i;
t15 = t2.*(8.1e+1./1.0e+3);
t16 = t3.*(8.1e+1./1.0e+3);
t17 = t4.*(8.1e+1./1.0e+3);
t18 = t5.*(8.1e+1./1.0e+3);
t21 = t4.*8.1e-2i;
t22 = t5.*8.1e-2i;
t10 = -t6;
t11 = -t9;
t14 = -t12;
t19 = -t15;
t20 = -t18;
t23 = -t21;
t24 = t8+t11;
t26 = t7+t10+3.0./2.0e+1;
t28 = t17+t20;
t30 = t16+t19+8.1e+1./1.0e+3;
t25 = t24.^2;
t27 = t26.^2;
t29 = t28.^2;
t31 = t30.^2;
t32 = t25+t27;
t33 = t32.^2;
t34 = -t33;
t35 = t29+t31+t34;
t36 = sqrt(t35);
t37 = t36.*1i;
t38 = t22+t23+t30+t32+t37;
t39 = angle(t38);
t40 = t39.*2.0;
t41 = -t40;
t42 = cos(t40);
t43 = sin(t40);
t44 = phi1+t41;
t45 = phi4+t41;
t48 = t42.*(2.7e+1./1.0e+2);
t49 = t43.*(2.7e+1./1.0e+2);
t51 = t43.*2.7e-1i;
t46 = sin(t44);
t47 = sin(t45);
t50 = -t48;
t52 = -t51;
t53 = t8+t49;
t55 = t6+t48-3.0./4.0e+1;
t54 = t53.^2;
t56 = t55.^2;
t57 = t12+t51+t55;
t64 = t13+t14+t26+t50+t52;
t58 = angle(t57);
t59 = t54+t56;
t65 = angle(t64);
t60 = -t58;
t63 = 1.0./sqrt(t59);
t66 = -t65;
t61 = phi1+t60;
t62 = phi4+t60;
t67 = phi1+t66;
t68 = phi4+t66;
t71 = t40+t60;
t74 = t40+t66;
t77 = t60+t65;
t69 = sin(t67);
t70 = sin(t68);
t72 = cos(t71);
t73 = sin(t71);
t75 = sin(t74);
t78 = cos(t77);
t79 = sin(t77);
t76 = 1.0./t75;
T = [F.*(sin(t61).*(-3.0./2.0e+1)+t46.*t76.*t79.*(3.0./2.0e+1)+t69.*t73.*t76.*(3.0./2.0e+1))-Tp.*t63.*(cos(t61).*(-3.0./2.0e+1)+t46.*t76.*t78.*(3.0./2.0e+1)+t69.*t72.*t76.*(3.0./2.0e+1));-F.*(sin(t62).*(3.0./2.0e+1)+t47.*t76.*t79.*(3.0./2.0e+1)+t70.*t73.*t76.*(3.0./2.0e+1))+Tp.*t63.*(cos(t62).*(3.0./2.0e+1)+t47.*t76.*t78.*(3.0./2.0e+1)+t70.*t72.*t76.*(3.0./2.0e+1))];
end
